simulink model "Semi_DP_1Hz"  (Simulink 8.7)
settings: Solver=ode4  StartTime=0.0  StopTime=12600  FixedStep=1  RelTol=1e-3
PreLoadFcn:
  | load('Initialization_data.mat');
undefined symbols (not defined in the file or in its folder): D, M, Ma, magnitude, P_mean, QTF_Dir, QTF_Freq, QTF_P, QTF_P1, QTF_Phase, QTF_T, RAO_Amp, RAO_Dir, RAO_Freq, RAO_Phase, RAO_Vel
libraries: simulink_extras x5, simulink x3
(part 1 of 2)
settings Model: Creator=Lither  LastModifiedBy=Administrator
settings OptimizationCC: ExpressionDepthLimit=2147483647
settings DebuggingCC: FcnCallInpInsideContextMsg=EnableAllAsWarning  StateNameClashWarn=warning
settings GRTTargetCC: CombineOutputUpdateFcns=off  GRTInterface=on
settings ConfigComp: CovSFcnEnable=off

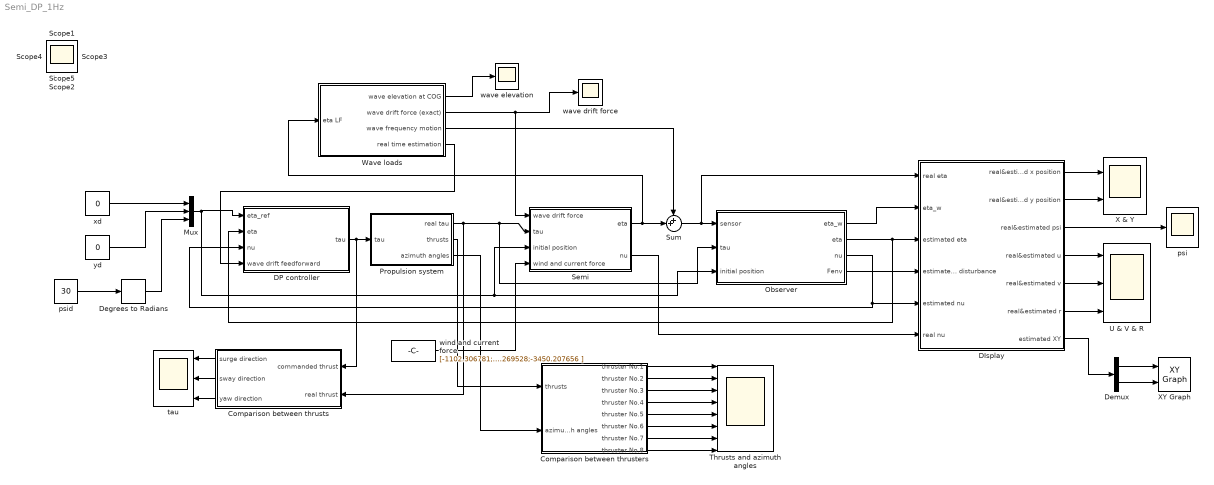
== system Semi_DP_1Hz ==
  Comparison between thrusters : Subsystem
  Comparison between thrusts : Subsystem
  DIsplay : Subsystem
  DP controller : Subsystem  mask(Nonlinear DP Controller){Kp=0.0015, Kd=0.06, Ki=1e-5, WFF_gain=0}
      mask prompts: Kp "Proportional Gain Matrix: Kp"; Kd "Derivative Gain Matrix: Kd"; Ki "Integral Gain Matrix: Ki"; WFF_gain "Wave feedforward Gain"
      mask help: PID controller for Set-Point Reulation in Surge, Sway and Yaw
      mask Help:
      | The nonlinear  PID controller uses the rotation matrix in yaw for proper scaling of the surge, sway and yaw gains as a function of the yaw angle.
      | INPUTS: (1) eta_ref, (2) eta, (3) nu. OUPUTS: (1) tau.
      mask Display: disp('PID controller')
  Degrees to Radians : simulink_extras/Transformations/Degrees to Radians
  Demux : Demux  Outputs=2
  Mux : Mux  Inputs=3
  Observer : Subsystem  mask(wave spectrum damping ratio){lambda=[0.0889 0.0839 0.1], w_o=[0.46 0.46 0.47], K3=5e5*diag([2 2 3500]), K4=6e5*diag([2 2 3500]), w_c=0.6, T=diag([10 10 10])}
      mask prompts: lambda "Relative damping ratio of wave spectrum: lambda"; w_o "Peak frequency of response spectrum: w_o (rad/s)"; K3 "Bias observer gain: K3"; K4 "Bias observer gain: K4"; w_c "Filter cut-off frequency: w_c (rad/s)"; T "Bias time constant: T (s)"
      mask init:
      | Zeta = 1;
      | Aw = blkdiag([0 1;-w_o(1)^2 -2*lambda(1)*w_o(1)],...
      |              [0 1;-w_o(2)^2 -2*lambda(2)*w_o(2)],...
      |              [0 1;-w_o(3)^2 -2*lambda(3)*w_o(3)]);
      | K1 = zeros(6,3);
      | for i =1:3
      |     K1(2*i-1,i) = -2*(Zeta - lambda(i))*w_c/w_o(i);
      |     K1(2*i,i) = 2*w_o(i)*(Zeta - lambda(i));
      | end
      | K2 = diag([w_c,w_c,w_c]);
      | Cw = zeros(3,6);
      | Cw(1,2) = 1;Cw(2,4) = 1;Cw(3,6) = 1;
      mask Display: disp('nonlinear passive observer')
  Propulsion system : Subsystem  mask{f0=[200;200;200;200;200;200;200;200], a0=[0;0;0;0;0;0;0;0], u0=[1; 1; 1; 1; 1; 1; 1; 1], wa=on}
      mask prompts: f0 "Initial values of thrusts"; a0 "Initial values of azimuth angles"; u0 "Thruster utilization"; wa "Show animation of thrust and azimuth angle"
  Semi : Subsystem  mask{wv=on}
      mask prompts: wv "Display animation of the vessel's motion"
  Sum : Sum  Inputs=++|
  Thrusts and azimuth angles : Scope  NumInputPorts=8
  U & V & R : Scope  NumInputPorts=3
  Wave loads : Subsystem
  X & Y : Scope  NumInputPorts=2
  XY Graph : simulink/Sinks/XY Graph  xmin=-20  xmax=20  ymin=-20  ymax=20  st=-1
  psi : Scope
  psid : Constant  Value=30
  tau : Scope  NumInputPorts=3
  wave drift force : Scope
  wave elevation : Scope
  wind and current force : Constant  Value=|
      | [-1102.306781;1391.269528;-3450.207656
      | ]
  xd : Constant  Value=0
  yd : Constant  Value=0
  Scope{,1..5} (6 alike) : Scope
  wires:
  xd/1 -> Mux/1
  yd/1 -> Mux/2
  Mux/1 -> Observer/3(initial position), Semi/3(initial position), DP controller/1(eta_ref)
  Semi/1(eta) -> Sum/2, Wave loads/1(eta LF)
  DP controller/1(tau) -> Propulsion system/1(tau), Comparison between thrusts/1(commanded thrust)
  Wave loads/2(wave drift force (exact)) -> Semi/1(wave drift force), wave drift force/1
  psid/1 -> Degrees to Radians/1
  Degrees to Radians/1 -> Mux/3
  Observer/3(nu) -> DP controller/3(nu), DIsplay/5(estimated nu)
  Observer/2(eta) -> DIsplay/3(estimated eta), DP controller/2(eta)
  Propulsion system/1(real tau) -> Comparison between thrusts/2(real thrust), Observer/2(tau), Semi/2(tau)
  Wave loads/1(wave elevation at COG) -> wave elevation/1
  Wave loads/3(wave frequency motion) -> Sum/1
  Sum/1 -> Observer/1(sensor), DIsplay/1(real eta)
  Comparison between thrusts/1(surge direction) -> tau/1
  Comparison between thrusts/2(sway direction) -> tau/2
  Comparison between thrusts/3(yaw direction) -> tau/3
  Propulsion system/2(thrusts) -> Comparison between thrusters/1(" thrusts")
  Propulsion system/3(azimuth angles) -> Comparison between thrusters/2(azimuth angles)
  Semi/2(nu) -> DIsplay/6(real nu)
  Observer/4(Fenv) -> DIsplay/4(estimated disturbance)
  DIsplay/1(real&estimated x position) -> X & Y/1
  DIsplay/2(real&estimated y position) -> X & Y/2
  DIsplay/3(real&estimated psi) -> psi/1
  DIsplay/4(real&estimated u) -> U & V & R/1
  DIsplay/5(real&estimated v) -> U & V & R/2
  Observer/1(eta_w) -> DIsplay/2(eta_w)
  DIsplay/6(real&estimated r) -> U & V & R/3
  wind and current force/1 -> Semi/4(wind and current force)
  Comparison between thrusters/1(thruster No.1) -> Thrusts and azimuth angles/1
  Comparison between thrusters/2(thruster No.2) -> Thrusts and azimuth angles/2
  Comparison between thrusters/8(thruster No.8) -> Thrusts and azimuth angles/8
  Comparison between thrusters/4(thruster No.4) -> Thrusts and azimuth angles/4
  Comparison between thrusters/6(thruster No.6) -> Thrusts and azimuth angles/6
  Comparison between thrusters/5(thruster No.5) -> Thrusts and azimuth angles/5
  Comparison between thrusters/3(thruster No.3) -> Thrusts and azimuth angles/3
  Comparison between thrusters/7(thruster No.7) -> Thrusts and azimuth angles/7
  Wave loads/4(real time estimation) -> DP controller/4(wave drift feedforward)
  Demux/1 -> XY Graph/1
  Demux/2 -> XY Graph/2
  DIsplay/7(estimated XY) -> Demux/1

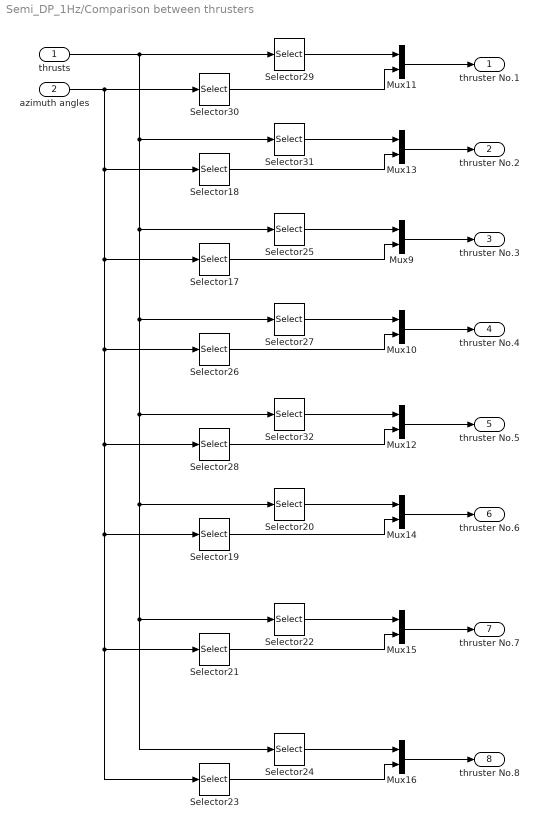
== system Semi_DP_1Hz/Comparison between thrusters ==
  " thrusts" : Inport
  azimuth angles : Inport  Port=2
  Mux{9..16} (8 alike) : Mux  Inputs=2
  Selector17 : Selector  InputPortWidth=8  IndexOptions=Index vector (dialog)  Indices=[3]  OutputSizes=1
  Selector18 : Selector  InputPortWidth=8  IndexOptions=Index vector (dialog)  Indices=[2]  OutputSizes=1
  Selector19 : Selector  InputPortWidth=8  IndexOptions=Index vector (dialog)  Indices=[6]  OutputSizes=1
  Selector20 : Selector  InputPortWidth=8  IndexOptions=Index vector (dialog)  Indices=[6]  OutputSizes=1
  Selector21 : Selector  InputPortWidth=8  IndexOptions=Index vector (dialog)  Indices=[7]  OutputSizes=1
  Selector22 : Selector  InputPortWidth=8  IndexOptions=Index vector (dialog)  Indices=[7]  OutputSizes=1
  Selector23 : Selector  InputPortWidth=8  IndexOptions=Index vector (dialog)  Indices=[8]  OutputSizes=1
  Selector24 : Selector  InputPortWidth=8  IndexOptions=Index vector (dialog)  Indices=[8]  OutputSizes=1
  Selector25 : Selector  InputPortWidth=8  IndexOptions=Index vector (dialog)  Indices=[3]  OutputSizes=1
  Selector26 : Selector  InputPortWidth=8  IndexOptions=Index vector (dialog)  Indices=[4]  OutputSizes=1
  Selector27 : Selector  InputPortWidth=8  IndexOptions=Index vector (dialog)  Indices=[4]  OutputSizes=1
  Selector28 : Selector  InputPortWidth=8  IndexOptions=Index vector (dialog)  Indices=[5]  OutputSizes=1
  Selector29 : Selector  InputPortWidth=8  IndexOptions=Index vector (dialog)  Indices=[1]  OutputSizes=1
  Selector30 : Selector  InputPortWidth=8  IndexOptions=Index vector (dialog)  Indices=[1]  OutputSizes=1
  Selector31 : Selector  InputPortWidth=8  IndexOptions=Index vector (dialog)  Indices=[2]  OutputSizes=1
  Selector32 : Selector  InputPortWidth=8  IndexOptions=Index vector (dialog)  Indices=[5]  OutputSizes=1
  thruster No.1 : Outport
  thruster No.2 : Outport  Port=2
  thruster No.3 : Outport  Port=3
  thruster No.4 : Outport  Port=4
  thruster No.5 : Outport  Port=5
  thruster No.6 : Outport  Port=6
  thruster No.7 : Outport  Port=7
  thruster No.8 : Outport  Port=8
  wires:
  Mux11/1 -> thruster No.1/1
  Selector29/1 -> Mux11/1
  Selector30/1 -> Mux11/2
  Selector31/1 -> Mux13/1
  Selector18/1 -> Mux13/2
  Mux13/1 -> thruster No.2/1
  " thrusts"/1 -> Selector29/1, Selector31/1, Selector25/1, Selector27/1, Selector32/1, Selector20/1, Selector22/1, Selector24/1
  Selector25/1 -> Mux9/1
  Selector17/1 -> Mux9/2
  Mux9/1 -> thruster No.3/1
  Selector27/1 -> Mux10/1
  Selector26/1 -> Mux10/2
  Selector32/1 -> Mux12/1
  Selector28/1 -> Mux12/2
  Selector20/1 -> Mux14/1
  Selector19/1 -> Mux14/2
  Mux10/1 -> thruster No.4/1
  Mux12/1 -> thruster No.5/1
  Mux14/1 -> thruster No.6/1
  azimuth angles/1 -> Selector30/1, Selector18/1, Selector17/1, Selector26/1, Selector28/1, Selector19/1, Selector23/1, Selector21/1
  Selector22/1 -> Mux15/1
  Selector21/1 -> Mux15/2
  Mux15/1 -> thruster No.7/1
  Selector24/1 -> Mux16/1
  Selector23/1 -> Mux16/2
  Mux16/1 -> thruster No.8/1

== system Semi_DP_1Hz/Comparison between thrusts ==
  commanded thrust : Inport
  real thrust : Inport  Port=2
  Mux3 : Mux  Inputs=2
  Mux5 : Mux  Inputs=2
  Mux6 : Mux  Inputs=2
  Selector10 : Selector  InputPortWidth=3  IndexOptions=Index vector (dialog)  Indices=[2]  OutputSizes=1
  Selector11 : Selector  InputPortWidth=3  IndexOptions=Index vector (dialog)  Indices=[3]  OutputSizes=1
  Selector6 : Selector  InputPortWidth=3  IndexOptions=Index vector (dialog)  Indices=[1]  OutputSizes=1
  Selector7 : Selector  InputPortWidth=3  IndexOptions=Index vector (dialog)  Indices=[1]  OutputSizes=1
  Selector8 : Selector  InputPortWidth=3  IndexOptions=Index vector (dialog)  Indices=[2]  OutputSizes=1
  Selector9 : Selector  InputPortWidth=3  IndexOptions=Index vector (dialog)  Indices=[3]  OutputSizes=1
  surge direction : Outport
  sway direction : Outport  Port=2
  yaw direction : Outport  Port=3
  wires:
  Selector9/1 -> Mux6/1
  Selector11/1 -> Mux6/2
  Selector10/1 -> Mux5/2
  Selector8/1 -> Mux5/1
  Selector7/1 -> Mux3/2
  Selector6/1 -> Mux3/1
  Mux3/1 -> surge direction/1
  Mux5/1 -> sway direction/1
  Mux6/1 -> yaw direction/1
  commanded thrust/1 -> Selector6/1, Selector8/1, Selector9/1
  real thrust/1 -> Selector7/1, Selector10/1, Selector11/1

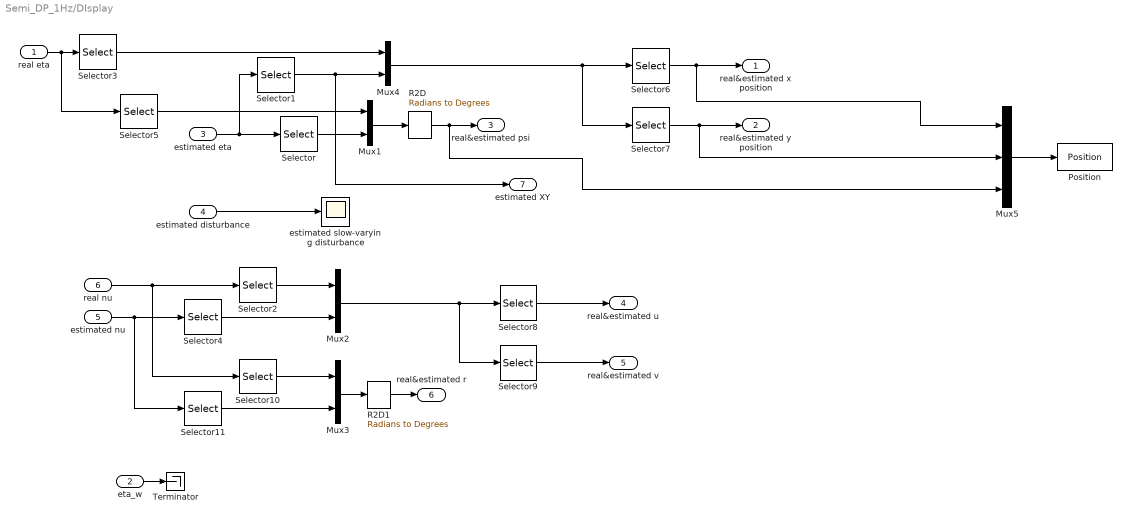
== system Semi_DP_1Hz/DIsplay ==
  real eta : Inport
  eta_w : Inport  Port=2
  estimated eta : Inport  Port=3
  estimated disturbance : Inport  Port=4
  estimated nu : Inport  Port=5
  real nu : Inport  Port=6
  Mux{1..4} (4 alike) : Mux  Inputs=2
  Mux5 : Mux  Inputs=3
  Position : ToWorkspace  VariableName=Position  SampleTime=-1
  R2D : simulink_extras/Transformations/Radians to Degrees
  R2D1 : simulink_extras/Transformations/Radians to Degrees
  Selector{,5,10..11} (4 alike) : Selector  InputPortWidth=3  IndexOptions=Index vector (dialog)  Indices=[3]  OutputSizes=1
  Selector{1..4} (4 alike) : Selector  InputPortWidth=3  IndexOptions=Index vector (dialog)  Indices=[1 2]  OutputSizes=1
  Selector6 : Selector  InputPortWidth=4  IndexOptions=Index vector (dialog)  Indices=[1 3]  OutputSizes=1
  Selector7 : Selector  InputPortWidth=4  IndexOptions=Index vector (dialog)  Indices=[2 4]  OutputSizes=1
  Selector8 : Selector  InputPortWidth=4  IndexOptions=Index vector (dialog)  Indices=[1 3]  OutputSizes=1
  Selector9 : Selector  InputPortWidth=4  IndexOptions=Index vector (dialog)  Indices=[2 4]  OutputSizes=1
  Terminator : Terminator
  estimated slow-varying disturbance : Scope
  real&estimated x position : Outport
  real&estimated y position : Outport  Port=2
  real&estimated psi : Outport  Port=3
  real&estimated u : Outport  Port=4
  real&estimated v : Outport  Port=5
  real&estimated r : Outport  Port=6
  estimated XY : Outport  Port=7
  wires:
  Selector/1 -> Mux1/2
  Mux1/1 -> R2D/1
  Selector1/1 -> estimated XY/1, Mux4/2
  Selector5/1 -> Mux1/1
  Selector2/1 -> Mux2/1
  Selector4/1 -> Mux2/2
  real eta/1 -> Selector3/1, Selector5/1
  estimated eta/1 -> Selector/1, Selector1/1
  real nu/1 -> Selector2/1, Selector10/1
  eta_w/1 -> Terminator/1
  estimated disturbance/1 -> estimated slow-varying disturbance/1
  Mux2/1 -> Selector8/1, Selector9/1
  estimated nu/1 -> Selector4/1, Selector11/1
  Mux4/1 -> Selector6/1, Selector7/1
  Selector8/1 -> real&estimated u/1
  Selector9/1 -> real&estimated v/1
  Mux3/1 -> R2D1/1
  R2D1/1 -> real&estimated r/1
  Selector10/1 -> Mux3/1
  Selector11/1 -> Mux3/2
  Selector3/1 -> Mux4/1
  R2D/1 -> Mux5/3, real&estimated psi/1
  Selector6/1 -> Mux5/1, real&estimated x position/1
  Selector7/1 -> Mux5/2, real&estimated y position/1
  Mux5/1 -> Position/1

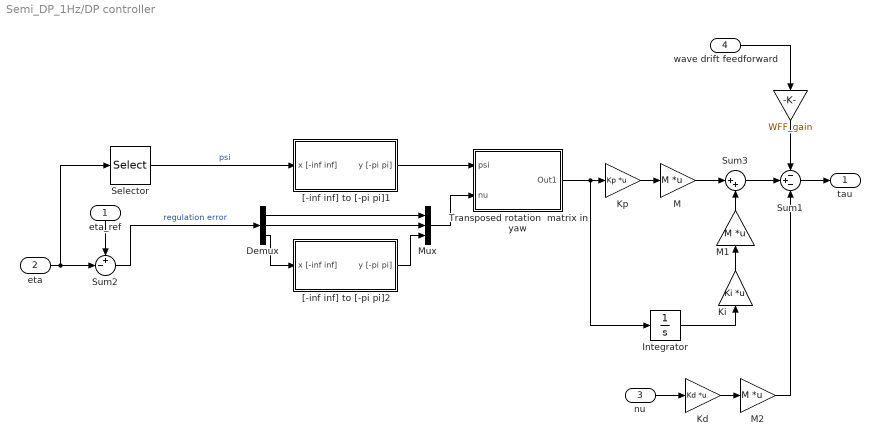
== system Semi_DP_1Hz/DP controller ==
  eta_ref : Inport
  eta : Inport  Port=2
  nu : Inport  Port=3
  wave drift feedforward : Inport  Port=4
  " " : Gain  Gain=WFF_gain  SaturateOnIntegerOverflow=on  OutDataTypeStr=Inherit: Same as input  ParamDataTypeStr=Inherit: Same as input
  Demux : Demux  Outputs=3
  Integrator : Integrator
  Kd : Gain  Gain=Kd  Multiplication=Matrix(K*u)  SaturateOnIntegerOverflow=on  OutDataTypeStr=Inherit: Same as input  ParamDataTypeStr=Inherit: Same as input
  Ki : Gain  Gain=Ki  Multiplication=Matrix(K*u)  SaturateOnIntegerOverflow=on  OutDataTypeStr=Inherit: Same as input  ParamDataTypeStr=Inherit: Same as input
  Kp : Gain  Gain=Kp  Multiplication=Matrix(K*u)  SaturateOnIntegerOverflow=on  OutDataTypeStr=Inherit: Same as input  ParamDataTypeStr=Inherit: Same as input
  M : Gain  Gain=M  Multiplication=Matrix(K*u)  SaturateOnIntegerOverflow=on  OutDataTypeStr=Inherit: Same as input  ParamDataTypeStr=Inherit: Same as input
  M1 : Gain  Gain=M  Multiplication=Matrix(K*u)  SaturateOnIntegerOverflow=on  OutDataTypeStr=Inherit: Same as input  ParamDataTypeStr=Inherit: Same as input
  M2 : Gain  Gain=M  Multiplication=Matrix(K*u)  SaturateOnIntegerOverflow=on  OutDataTypeStr=Inherit: Same as input  ParamDataTypeStr=Inherit: Same as input
  Mux : Mux  Inputs=3
  Selector : Selector  InputPortWidth=3  IndexOptions=Index vector (dialog)  Indices=[ 3]  OutputSizes=1
  Sum1 : Sum  Inputs=-+-  SaturateOnIntegerOverflow=on  InputSameDT=on  OutDataTypeStr=Inherit: Same as first input
  Sum2 : Sum  Inputs=+-|  SaturateOnIntegerOverflow=on  InputSameDT=on  OutDataTypeStr=Inherit: Same as first input
  Sum3 : Sum  Inputs=|++  SaturateOnIntegerOverflow=on  InputSameDT=on  OutDataTypeStr=Inherit: Same as first input
  Transposed rotation  matrix in yaw : Subsystem
  "[-inf inf] to [-pi pi]1" : Subsystem
  "[-inf inf] to [-pi pi]2" : Subsystem
  tau : Outport  InitialOutput=0
  wires:
  "[-inf inf] to [-pi pi]1"/1(y [-pi pi]) -> Transposed rotation  matrix in yaw/1(psi)
  Selector/1 -> "[-inf inf] to [-pi pi]1"/1(x [-inf inf])  "psi"
  Mux/1 -> Transposed rotation  matrix in yaw/2(nu)
  Demux/1 -> Mux/1
  Demux/2 -> Mux/2
  "[-inf inf] to [-pi pi]2"/1(y [-pi pi]) -> Mux/3
  Sum2/1 -> Demux/1  "regulation error"
  Demux/3 -> "[-inf inf] to [-pi pi]2"/1(x [-inf inf])
  eta_ref/1 -> Sum2/1
  Sum1/1 -> tau/1
  eta/1 -> Sum2/2, Selector/1
  nu/1 -> Kd/1
  Integrator/1 -> Ki/1
  Kp/1 -> M/1
  Ki/1 -> M1/1
  Transposed rotation  matrix in yaw/1(Out1) -> Kp/1, Integrator/1
  Kd/1 -> M2/1
  M/1 -> Sum3/1
  M1/1 -> Sum3/2
  wave drift feedforward/1 -> " "/1
  " "/1 -> Sum1/1
  M2/1 -> Sum1/3
  Sum3/1 -> Sum1/2

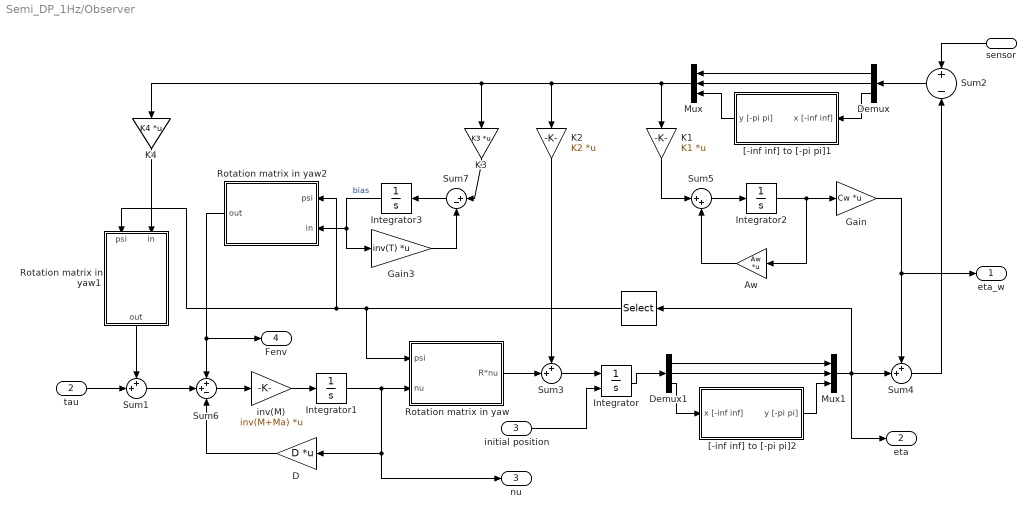
== system Semi_DP_1Hz/Observer ==
  sensor : Inport
  tau : Inport  Port=2
  initial position : Inport  Port=3
  " " : Selector  InputPortWidth=3  IndexOptions=Index vector (dialog)  Indices=[3]  OutputSizes=1
  Aw : Gain  Gain=Aw  Multiplication=Matrix(K*u)  SaturateOnIntegerOverflow=on  OutDataTypeStr=Inherit: Same as input  ParamDataTypeStr=Inherit: Same as input
  D : Gain  Gain=D  Multiplication=Matrix(K*u)  SaturateOnIntegerOverflow=on  OutDataTypeStr=Inherit: Same as input  ParamDataTypeStr=Inherit: Same as input
  Demux : Demux  Outputs=3
  Demux1 : Demux  Outputs=3
  Gain : Gain  Gain=Cw  Multiplication=Matrix(K*u)
  Gain3 : Gain  Gain=inv(T)  Multiplication=Matrix(K*u)  SaturateOnIntegerOverflow=on  OutDataTypeStr=Inherit: Same as input  ParamDataTypeStr=Inherit: Same as input
  Integrator : Integrator  InitialConditionSource=external
  Integrator1 : Integrator
  Integrator2 : Integrator
  Integrator3 : Integrator
  K1 : Gain  Gain=K1  Multiplication=Matrix(K*u)  SaturateOnIntegerOverflow=on  OutDataTypeStr=Inherit: Same as input  ParamDataTypeStr=Inherit: Same as input
  K2 : Gain  Gain=K2  Multiplication=Matrix(K*u)  SaturateOnIntegerOverflow=on  OutDataTypeStr=Inherit: Same as input  ParamDataTypeStr=Inherit: Same as input
  K3 : Gain  Gain=K3  Multiplication=Matrix(K*u)  SaturateOnIntegerOverflow=on  OutDataTypeStr=Inherit: Same as input  ParamDataTypeStr=Inherit: Same as input
  K4 : Gain  Gain=K4  Multiplication=Matrix(K*u)  SaturateOnIntegerOverflow=on  OutDataTypeStr=Inherit: Same as input  ParamDataTypeStr=Inherit: Same as input
  Mux : Mux  Inputs=3
  Mux1 : Mux  Inputs=3
  Rotation matrix in yaw : Subsystem
  Rotation matrix in yaw1 : Subsystem
  Rotation matrix in yaw2 : Subsystem
  Sum1 : Sum  Inputs=++|  SaturateOnIntegerOverflow=on  InputSameDT=on  OutDataTypeStr=Inherit: Same as first input
  Sum2 : Sum  Inputs=+|-  SaturateOnIntegerOverflow=on  InputSameDT=on  OutDataTypeStr=Inherit: Same as first input
  Sum3 : Sum  Inputs=++|  SaturateOnIntegerOverflow=on  InputSameDT=on  OutDataTypeStr=Inherit: Same as first input
  Sum4 : Sum  Inputs=++|  SaturateOnIntegerOverflow=on  InputSameDT=on  OutDataTypeStr=Inherit: Same as first input
  Sum5 : Sum  Inputs=|++  SaturateOnIntegerOverflow=on  InputSameDT=on  OutDataTypeStr=Inherit: Same as first input
  Sum6 : Sum  Inputs=++-  SaturateOnIntegerOverflow=on  InputSameDT=on  OutDataTypeStr=Inherit: Same as first input
  Sum7 : Sum  Inputs=|+-  SaturateOnIntegerOverflow=on  InputSameDT=on  OutDataTypeStr=Inherit: Same as first input
  "[-inf inf] to [-pi pi]1" : Subsystem  mask([-inf inf] to [-pi pi]){}
      mask help: Converts an angle in rad to (-pi pi)
  "[-inf inf] to [-pi pi]2" : Subsystem
  inv(M) : Gain  Gain=inv(M+Ma)  Multiplication=Matrix(K*u)  SaturateOnIntegerOverflow=on  OutDataTypeStr=Inherit: Same as input  ParamDataTypeStr=Inherit: Same as input
  eta_w : Outport
  eta : Outport  Port=2
  nu : Outport  Port=3
  Fenv : Outport  Port=4
  wires:
  tau/1 -> Sum1/2
  sensor/1 -> Sum2/1
  Gain3/1 -> Sum7/2
  Sum7/1 -> Integrator3/1
  Integrator3/1 -> Gain3/1, Rotation matrix in yaw2/2(in)  "bias"
  Sum4/1 -> Sum2/2
  Integrator/1 -> Demux1/1
  Sum3/1 -> Integrator/1
  Sum2/1 -> Demux/1
  Demux/3 -> "[-inf inf] to [-pi pi]1"/1(x [-inf inf])
  "[-inf inf] to [-pi pi]1"/1(y [-pi pi]) -> Mux/3
  Demux/1 -> Mux/1
  Demux/2 -> Mux/2
  Mux/1 -> K1/1, K2/1, K4/1, K3/1
  Demux1/1 -> Mux1/1
  Demux1/2 -> Mux1/2
  "[-inf inf] to [-pi pi]2"/1(y [-pi pi]) -> Mux1/3
  Demux1/3 -> "[-inf inf] to [-pi pi]2"/1(x [-inf inf])
  Mux1/1 -> eta/1, Sum4/2, " "/1
  Sum5/1 -> Integrator2/1
  K1/1 -> Sum5/1
  Integrator2/1 -> Gain/1, Aw/1
  Aw/1 -> Sum5/2
  K2/1 -> Sum3/1
  Rotation matrix in yaw/1(R*nu) -> Sum3/2
  K3/1 -> Sum7/1
  inv(M)/1 -> Integrator1/1
  Sum6/1 -> inv(M)/1
  Integrator1/1 -> Rotation matrix in yaw/2(nu), D/1, nu/1
  " "/1 -> Rotation matrix in yaw/1(psi), Rotation matrix in yaw1/1(psi), Rotation matrix in yaw2/1(psi)
  Sum1/1 -> Sum6/2
  D/1 -> Sum6/3
  K4/1 -> Rotation matrix in yaw1/2(in)
  Rotation matrix in yaw1/1(out) -> Sum1/1
  Rotation matrix in yaw2/1(out) -> Sum6/1, Fenv/1
  initial position/1 -> Integrator/2
  Gain/1 -> Sum4/1, eta_w/1

== system Semi_DP_1Hz/Propulsion system ==
  tau : Inport
  AzimuthAngle : ToWorkspace  VariableName=AziAng  SampleTime=-1
  Gain : Gain  Gain=1/1000
  Gain1 : Gain  Gain=1000
  Level-2 MATLAB S-Function : M-S-Function  FunctionName=msfunTA_PA  Parameters=f0,a0,wa,u0
  RealTau : ToWorkspace  VariableName=RealTau  SampleTime=-1
  Terminator : Terminator
  Terminator1 : Terminator
  Terminator2 : Terminator
  ThrusterForce : ToWorkspace  VariableName=Thrust  SampleTime=-1
  real tau : Outport
  thrusts : Outport  Port=2
  azimuth angles : Outport  Port=3
  wires:
  tau/1 -> Gain/1
  Level-2 MATLAB S-Function/2 -> Terminator/1
  Level-2 MATLAB S-Function/3 -> AzimuthAngle/1, azimuth angles/1
  Level-2 MATLAB S-Function/4 -> Terminator1/1
  Level-2 MATLAB S-Function/5 -> Gain1/1
  Level-2 MATLAB S-Function/6 -> Terminator2/1
  Level-2 MATLAB S-Function/1 -> ThrusterForce/1, thrusts/1
  Gain/1 -> Level-2 MATLAB S-Function/1
  Gain1/1 -> RealTau/1, real tau/1

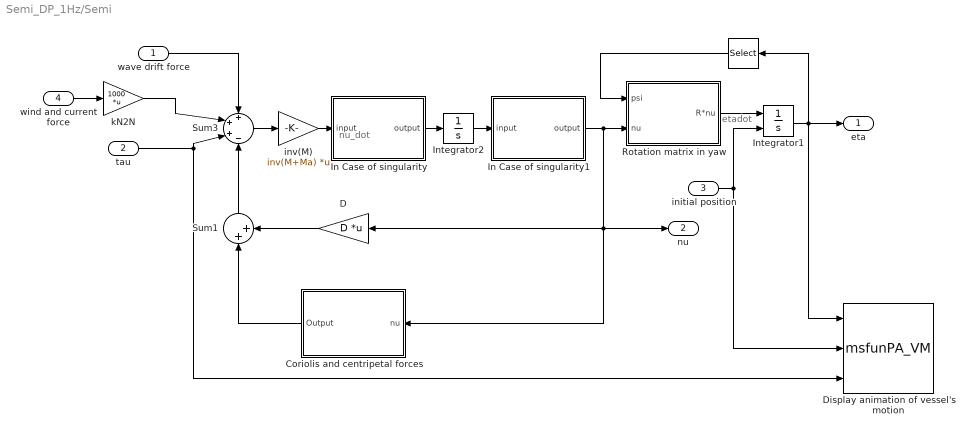
== system Semi_DP_1Hz/Semi ==
  note: nu_dot
  note: etadot
  wave drift force : Inport
  tau : Inport  Port=2
  initial position : Inport  Port=3
  wind and current force : Inport  Port=4
  " " : Selector  InputPortWidth=3  IndexOptions=Index vector (dialog)  Indices=[3]  OutputSizes=1
  Coriolis and centripetal forces : Subsystem
  D : Gain  Gain=D  Multiplication=Matrix(K*u)  SaturateOnIntegerOverflow=on  OutDataTypeStr=Inherit: Same as input  ParamDataTypeStr=Inherit: Same as input
  Display animation of vessel's motion : M-S-Function  FunctionName=msfunPA_VM  Parameters=wv
  In Case of singularity : Subsystem
  In Case of singularity1 : Subsystem
  Integrator1 : Integrator  InitialConditionSource=external  InitialCondition=1.05
  Integrator2 : Integrator
  Rotation matrix in yaw : Subsystem
  Sum1 : Sum  Inputs=|++  SaturateOnIntegerOverflow=on  InputSameDT=on  OutDataTypeStr=Inherit: Same as first input
  Sum3 : Sum  Inputs=+++-  SaturateOnIntegerOverflow=on  InputSameDT=on  OutDataTypeStr=Inherit: Same as first input
  inv(M) : Gain  Gain=inv(M+Ma)  Multiplication=Matrix(K*u)  SaturateOnIntegerOverflow=on  OutDataTypeStr=Inherit: Same as input  ParamDataTypeStr=Inherit: Same as input
  kN2N : Gain  Gain=1000  Multiplication=Matrix(K*u)  SaturateOnIntegerOverflow=on  OutDataTypeStr=Inherit: Same as input  ParamDataTypeStr=Inherit: Same as input
  eta : Outport
  nu : Outport  Port=2
  wires:
  Sum3/1 -> inv(M)/1
  inv(M)/1 -> In Case of singularity/1(input)
  Rotation matrix in yaw/1(R*nu) -> Integrator1/1
  Integrator1/1 -> eta/1, " "/1, Display animation of vessel's motion/1
  " "/1 -> Rotation matrix in yaw/1(psi)
  tau/1 -> Display animation of vessel's motion/3, Sum3/3
  initial position/1 -> Integrator1/2, Display animation of vessel's motion/2
  Sum1/1 -> Sum3/4
  wind and current force/1 -> kN2N/1
  Integrator2/1 -> In Case of singularity1/1(input)
  In Case of singularity/1(output) -> Integrator2/1
  In Case of singularity1/1(output) -> Rotation matrix in yaw/2(nu), D/1, Coriolis and centripetal forces/1(nu), nu/1
  wave drift force/1 -> Sum3/1
  D/1 -> Sum1/2
  Coriolis and centripetal forces/1(Output) -> Sum1/1
  kN2N/1 -> Sum3/2

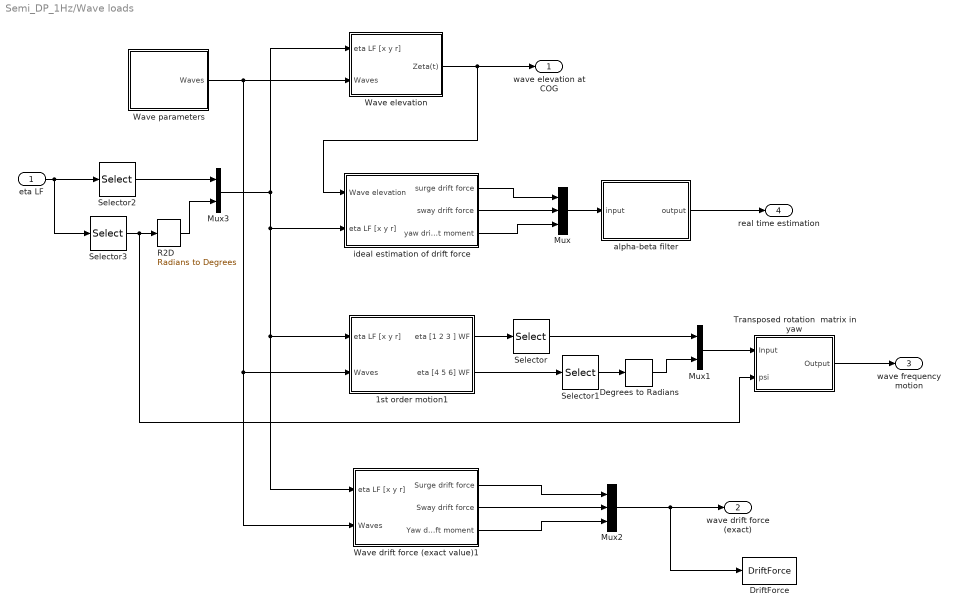
== system Semi_DP_1Hz/Wave loads ==
  eta LF : Inport
  1st order motion1 : Subsystem  mask(Motion RAO){}
      mask help: Calculate the wave-frequency motion of a vessel in 6 DOF from its RAOs and a sea state defined by a set of harmonic waves.
  Degrees to Radians : simulink_extras/Transformations/Degrees to Radians
  DriftForce : ToWorkspace  VariableName=DriftForce  SampleTime=-1
  Mux : Mux  Inputs=3
  Mux1 : Mux  Inputs=2
  Mux2 : Mux  Inputs=3
  Mux3 : Mux  Inputs=2
  R2D : simulink_extras/Transformations/Radians to Degrees
  Selector : Selector  InputPortWidth=3  IndexOptions=Index vector (dialog)  Indices=[1 2]  OutputSizes=1
  Selector1 : Selector  InputPortWidth=3  IndexOptions=Index vector (dialog)  Indices=[3]  OutputSizes=1
  Selector2 : Selector  InputPortWidth=3  IndexOptions=Index vector (dialog)  Indices=[1 2]  OutputSizes=1
  Selector3 : Selector  InputPortWidth=3  IndexOptions=Index vector (dialog)  Indices=[3]  OutputSizes=1
  Transposed rotation  matrix in yaw : Subsystem
  Wave drift force (exact value)1 : Subsystem  mask(Wave drift force (exact value based on full QTF matrix)){}
      mask help: Calculate the mean and slow varying wave drift forces based on full QTF matrix.
  Wave elevation : Subsystem  mask(Wave elevation){}
      mask help: Caclulates wave surface elevation Zeta at the point [x y].
  Wave parameters : Subsystem  mask(JONSWAP Spectrum Generator){Hs=5.27, Tp=13.4, gamma=3.3, nfr=200, displayplots=off, Zeta_a=0, Omega=0, Phase=0, Wavenum=0}
      mask prompts: Hs "Significant wave height Hs (m)"; Tp "Peak period (s)"; gamma "Spectrum peakedness factor"; nfr "Number of frequencies"; displayplots "Display plot"; Zeta_a "Amplitude vector 'Zeta_a' (m)"; Omega "Frequency vector 'Omega' (rad/s)"; Phase "Phase vector 'Phase' (rad)"; Wavenum "Wave number vector 'Wavenum' (1/m)"
      mask help: Generate long-crested irregular waves based on JONSWAP spectrum
      mask init:
      | [Omega,Zeta_a,Wavenum,Phase]=jonspec_fixed(Hs,Tp,gamma,nfr,displayplots);
  alpha-beta filter : Subsystem  mask(alpha-beta filter){a=8e-2, b=1e-12}
      mask prompts: a "alpha"; b "beta"
  "ideal estimation of drift force " : Subsystem  mask(Estimate the second order wave force in real time){}
      mask help: The real-time estimation of wave drift force is based on the mean value of QTF_P on the diagonal and wave elevation.
  wave elevation at COG : Outport
  wave drift force (exact) : Outport  Port=2
  wave frequency motion : Outport  Port=3
  real time estimation : Outport  Port=4
  wires:
  Wave elevation/1(Zeta(t)) -> "ideal estimation of drift force "/1(Wave elevation), wave elevation at COG/1
  Wave parameters/1(Waves) -> Wave elevation/2(Waves), Wave drift force (exact value)1/2(Waves), 1st order motion1/2(Waves)
  eta LF/1 -> Selector2/1, Selector3/1
  1st order motion1/1(eta [1 2 3 ] WF) -> Selector/1
  Selector/1 -> Mux1/1
  1st order motion1/2(eta [4 5 6] WF) -> Selector1/1
  Selector1/1 -> Degrees to Radians/1
  Mux1/1 -> Transposed rotation  matrix in yaw/1(Input)
  Wave drift force (exact value)1/2(Sway drift force) -> Mux2/2
  Wave drift force (exact value)1/3(Yaw drift moment) -> Mux2/3
  Wave drift force (exact value)1/1(Surge drift force) -> Mux2/1
  Selector3/1 -> R2D/1, Transposed rotation  matrix in yaw/2(psi)
  Selector2/1 -> Mux3/1
  R2D/1 -> Mux3/2
  Mux3/1 -> "ideal estimation of drift force "/2(eta LF [x y r]), Wave drift force (exact value)1/1(eta LF [x y r]), 1st order motion1/1(eta LF [x y r]), Wave elevation/1(eta LF [x y r])
  Degrees to Radians/1 -> Mux1/2
  Transposed rotation  matrix in yaw/1(Output) -> wave frequency motion/1
  "ideal estimation of drift force "/1(surge drift force) -> Mux/1
  "ideal estimation of drift force "/2(sway drift force) -> Mux/2
  Mux/1 -> alpha-beta filter/1(input)
  "ideal estimation of drift force "/3(yaw drift moment) -> Mux/3
  Mux2/1 -> DriftForce/1, wave drift force (exact)/1
  alpha-beta filter/1(output) -> real time estimation/1

== system Semi_DP_1Hz/DP controller/Transposed rotation  matrix in yaw ==
  psi : Inport
  nu : Inport  Port=2
  Mux : Mux  Inputs=2
  Mux1 : Mux  Inputs=3
  Row1 : Fcn  Expr=cos(u(1))*u(2)+sin(u(1))*u(3)
  Row2 : Fcn  Expr=-sin(u(1))*u(2)+cos(u(1))*u(3)
  Row3 : Fcn  Expr=u(4)
  Out1 : Outport
  wires:
  Mux/1 -> Row3/1, Row2/1, Row1/1
  Row1/1 -> Mux1/1
  Row2/1 -> Mux1/2
  Row3/1 -> Mux1/3
  Mux1/1 -> Out1/1
  psi/1 -> Mux/1
  nu/1 -> Mux/2

== system Semi_DP_1Hz/DP controller/[-inf inf] to [-pi pi]1 ==
  note: x
  note: r
  x [-inf inf] : Inport
  Constant : Constant  Value=2*pi
  Gain : Gain  Gain=pi  SaturateOnIntegerOverflow=on  OutDataTypeStr=Inherit: Same as input  ParamDataTypeStr=Inherit: Same as input
  Math Function : Math  Operator=rem  SaturateOnIntegerOverflow=on
  Saturation : Saturate  UpperLimit=1e10  LowerLimit=-1e10
  Sign : Signum
  Sum : Sum  Inputs=|+-  SaturateOnIntegerOverflow=on
  Sum1 : Sum  Inputs=|++  SaturateOnIntegerOverflow=on
  y [-pi pi] : Outport
  wires:
  x [-inf inf]/1 -> Saturation/1
  Sign/1 -> Gain/1
  Gain/1 -> Sum/2, Sum1/2
  Sum1/1 -> Math Function/1
  Constant/1 -> Math Function/2
  Math Function/1 -> Sum/1
  Sum/1 -> y [-pi pi]/1
  Saturation/1 -> Sum1/1, Sign/1

== system Semi_DP_1Hz/DP controller/[-inf inf] to [-pi pi]2 ==
  note: r
  note: x
  x [-inf inf] : Inport
  Constant : Constant  Value=2*pi
  Gain : Gain  Gain=pi  SaturateOnIntegerOverflow=on  OutDataTypeStr=Inherit: Same as input  ParamDataTypeStr=Inherit: Same as input
  Math Function : Math  Operator=rem  SaturateOnIntegerOverflow=on
  Saturation : Saturate  UpperLimit=1e10  LowerLimit=-1e10
  Sign : Signum
  Sum : Sum  Inputs=|+-  SaturateOnIntegerOverflow=on
  Sum1 : Sum  Inputs=|++  SaturateOnIntegerOverflow=on
  y [-pi pi] : Outport
  wires:
  Saturation/1 -> Sign/1, Sum1/1
  Sum/1 -> y [-pi pi]/1
  Math Function/1 -> Sum/1
  Constant/1 -> Math Function/2
  Sum1/1 -> Math Function/1
  Gain/1 -> Sum1/2, Sum/2
  Sign/1 -> Gain/1
  x [-inf inf]/1 -> Saturation/1

== system Semi_DP_1Hz/Observer/Rotation matrix in yaw ==
  psi : Inport
  nu : Inport  Port=2
  Fcn : Fcn  Expr=cos(u(1))*u(2)-sin(u(1))*u(3)
  Fcn1 : Fcn  Expr=sin(u(1))*u(2)+cos(u(1))*u(3)
  Fcn2 : Fcn  Expr=u(4)
  Mux : Mux  Inputs=2
  Mux1 : Mux  Inputs=3
  R*nu : Outport
  wires:
  Mux1/1 -> R*nu/1  "eta_dot"
  Mux/1 -> Fcn/1, Fcn1/1, Fcn2/1
  psi/1 -> Mux/1
  nu/1 -> Mux/2
  Fcn1/1 -> Mux1/2  "y_dot"
  Fcn/1 -> Mux1/1  "x_dot"
  Fcn2/1 -> Mux1/3  "psi_dot"

== system Semi_DP_1Hz/Observer/Rotation matrix in yaw1 ==
  psi : Inport
  in : Inport  Port=2
  Fcn : Fcn  Expr=cos(u(1))*u(2)+sin(u(1))*u(3)
  Fcn1 : Fcn  Expr=-sin(u(1))*u(2)+cos(u(1))*u(3)
  Fcn2 : Fcn  Expr=u(4)
  Mux : Mux  Inputs=2
  Mux1 : Mux  Inputs=3
  out : Outport
  wires:
  Fcn2/1 -> Mux1/3
  Fcn/1 -> Mux1/1
  Fcn1/1 -> Mux1/2
  in/1 -> Mux/2
  psi/1 -> Mux/1
  Mux/1 -> Fcn2/1, Fcn1/1, Fcn/1
  Mux1/1 -> out/1

== system Semi_DP_1Hz/Observer/Rotation matrix in yaw2 ==
  psi : Inport
  in : Inport  Port=2
  Fcn : Fcn  Expr=cos(u(1))*u(2)+sin(u(1))*u(3)
  Fcn1 : Fcn  Expr=-sin(u(1))*u(2)+cos(u(1))*u(3)
  Fcn2 : Fcn  Expr=u(4)
  Mux : Mux  Inputs=2
  Mux1 : Mux  Inputs=3
  out : Outport
  wires:
  Mux1/1 -> out/1
  Mux/1 -> Fcn/1, Fcn1/1, Fcn2/1
  psi/1 -> Mux/1
  in/1 -> Mux/2
  Fcn1/1 -> Mux1/2
  Fcn/1 -> Mux1/1
  Fcn2/1 -> Mux1/3

== system Semi_DP_1Hz/Observer/[-inf inf] to [-pi pi]1 ==
  note: x
  note: r
  x [-inf inf] : Inport
  Constant : Constant  Value=2*pi
  Gain : Gain  Gain=pi  SaturateOnIntegerOverflow=on  OutDataTypeStr=Inherit: Same as input  ParamDataTypeStr=Inherit: Same as input
  Math Function : Math  Operator=rem  SaturateOnIntegerOverflow=on
  Saturation : Saturate  UpperLimit=1e10  LowerLimit=-1e10
  Sign : Signum
  Sum : Sum  Inputs=|+-  SaturateOnIntegerOverflow=on
  Sum1 : Sum  Inputs=|++  SaturateOnIntegerOverflow=on
  y [-pi pi] : Outport
  wires:
  x [-inf inf]/1 -> Saturation/1
  Sign/1 -> Gain/1
  Gain/1 -> Sum/2, Sum1/2
  Sum1/1 -> Math Function/1
  Constant/1 -> Math Function/2
  Math Function/1 -> Sum/1
  Sum/1 -> y [-pi pi]/1
  Saturation/1 -> Sum1/1, Sign/1

== system Semi_DP_1Hz/Observer/[-inf inf] to [-pi pi]2 ==
  note: r
  note: x
  x [-inf inf] : Inport
  Constant : Constant  Value=2*pi
  Gain : Gain  Gain=pi  SaturateOnIntegerOverflow=on  OutDataTypeStr=Inherit: Same as input  ParamDataTypeStr=Inherit: Same as input
  Math Function : Math  Operator=rem  SaturateOnIntegerOverflow=on
  Saturation : Saturate  UpperLimit=1e10  LowerLimit=-1e10
  Sign : Signum
  Sum : Sum  Inputs=|+-  SaturateOnIntegerOverflow=on
  Sum1 : Sum  Inputs=|++  SaturateOnIntegerOverflow=on
  y [-pi pi] : Outport
  wires:
  Saturation/1 -> Sign/1, Sum1/1
  Sum/1 -> y [-pi pi]/1
  Math Function/1 -> Sum/1
  Constant/1 -> Math Function/2
  Sum1/1 -> Math Function/1
  Gain/1 -> Sum1/2, Sum/2
  Sign/1 -> Gain/1
  x [-inf inf]/1 -> Saturation/1

== system Semi_DP_1Hz/Semi/Coriolis and centripetal forces ==
  nu : Inport
  Mux : Mux  Inputs=3
  Selector1 : Selector  InputPortWidth=3  IndexOptions=Index vector (dialog)  Indices=[1 ]  OutputSizes=1
  Selector2 : Selector  InputPortWidth=3  IndexOptions=Index vector (dialog)  Indices=[2]  OutputSizes=1
  Selector3 : Selector  InputPortWidth=3  IndexOptions=Index vector (dialog)  Indices=[3]  OutputSizes=1
  Subsystem : Subsystem
  Subsystem1 : Subsystem
  Subsystem2 : Subsystem
  Output : Outport
  wires:
  nu/1 -> Selector1/1, Selector2/1, Selector3/1
  Selector2/1 -> Subsystem/1(v), Subsystem2/2(v)  "v"
  Selector3/1 -> Subsystem/2(r), Subsystem1/2(r), Subsystem2/3(r)  "r"
  Selector1/1 -> Subsystem1/1(u), Subsystem2/1(u)  "u"
  Subsystem/1(x direction) -> Mux/1
  Subsystem1/1(y direction) -> Mux/2
  Subsystem2/1(yaw direction) -> Mux/3
  Mux/1 -> Output/1

== system Semi_DP_1Hz/Semi/In Case of singularity ==
  input : Inport
  Compare To Constant : simulink/Logic and Bit Operations/Compare To Constant  relop=>=  const=1e8  OutDataTypeStr=boolean
  Stop Simulation : Stop
  output : Outport
  wires:
  input/1 -> output/1, Compare To Constant/1
  Compare To Constant/1 -> Stop Simulation/1

== system Semi_DP_1Hz/Semi/In Case of singularity1 ==
  input : Inport
  Compare To Constant : simulink/Logic and Bit Operations/Compare To Constant  relop=>=  const=1e10  OutDataTypeStr=boolean
  Stop Simulation : Stop
  output : Outport
  wires:
  input/1 -> output/1, Compare To Constant/1
  Compare To Constant/1 -> Stop Simulation/1

== system Semi_DP_1Hz/Semi/Rotation matrix in yaw ==
  psi : Inport
  nu : Inport  Port=2
  Fcn : Fcn  Expr=cos(u(1))*u(2)-sin(u(1))*u(3)
  Fcn1 : Fcn  Expr=sin(u(1))*u(2)+cos(u(1))*u(3)
  Fcn2 : Fcn  Expr=u(4)
  Mux : Mux  Inputs=2
  Mux1 : Mux  Inputs=3
  R*nu : Outport
  wires:
  Mux1/1 -> R*nu/1  "eta_dot"
  Mux/1 -> Fcn/1, Fcn1/1, Fcn2/1
  psi/1 -> Mux/1
  nu/1 -> Mux/2
  Fcn1/1 -> Mux1/2  "y_dot"
  Fcn/1 -> Mux1/1  "x_dot"
  Fcn2/1 -> Mux1/3  "psi_dot"

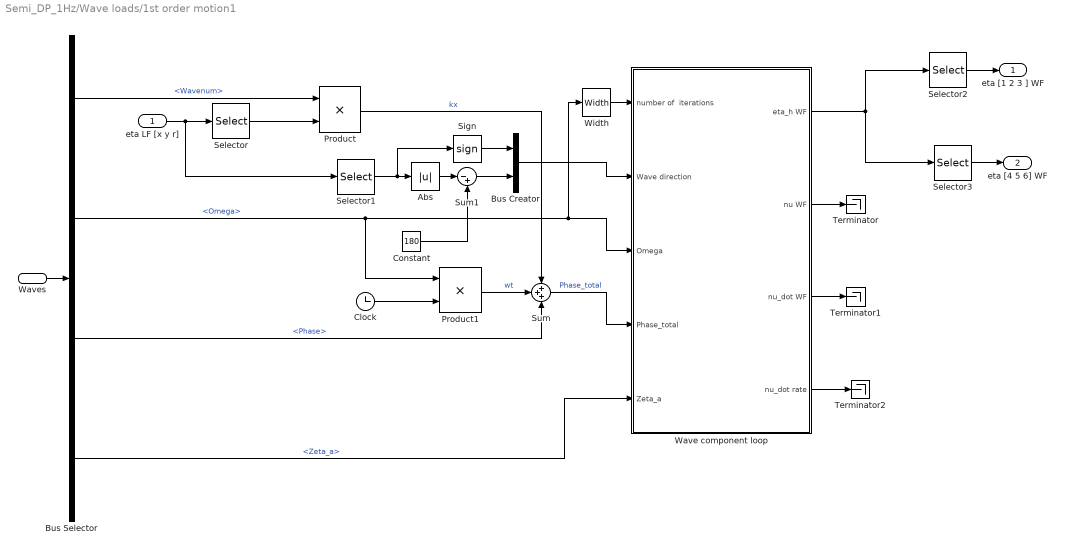
== system Semi_DP_1Hz/Wave loads/1st order motion1 ==
  eta LF [x y r] : Inport
  Waves : Inport  Port=2
  Abs : Abs
  Bus Creator : BusCreator  Inputs=2
  Bus Selector : BusSelector  OutputSignals=Wavenum,Omega,Phase,Zeta_a
  Clock : Clock
  Constant : Constant  Value=180
  Product : Product  Inputs=**  SaturateOnIntegerOverflow=on  OutDataTypeStr=Inherit: Same as first input
  Product1 : Product  Inputs=**  SaturateOnIntegerOverflow=on  OutDataTypeStr=Inherit: Same as first input
  Selector : Selector  InputPortWidth=3  IndexOptions=Index vector (dialog)  Indices=1  OutputSizes=1
  Selector1 : Selector  InputPortWidth=3  IndexOptions=Index vector (dialog)  Indices=3  OutputSizes=1
  Selector2 : Selector  InputPortWidth=6  IndexOptions=Index vector (dialog)  Indices=[1 2 3]  OutputSizes=1
  Selector3 : Selector  InputPortWidth=6  IndexOptions=Index vector (dialog)  Indices=[4 5 6]  OutputSizes=1
  Sign : Signum
  Sum : Sum  Inputs=+++  SaturateOnIntegerOverflow=on
  Sum1 : Sum  Inputs=|-+
  Terminator : Terminator
  Terminator1 : Terminator
  Terminator2 : Terminator
  Wave component loop : Subsystem  TreatAsAtomicUnit=on
  Width : Width  DataType=int32
  eta [1 2 3 ] WF : Outport
  eta [4 5 6] WF : Outport  Port=2
  wires:
  Wave component loop/1(eta_h WF) -> Selector2/1, Selector3/1
  Selector3/1 -> eta [4 5 6] WF/1
  Bus Creator/1 -> Wave component loop/2(Wave direction)
  Sum1/1 -> Bus Creator/2
  Sign/1 -> Bus Creator/1
  Abs/1 -> Sum1/1
  Selector1/1 -> Sign/1, Abs/1
  Constant/1 -> Sum1/2
  eta LF [x y r]/1 -> Selector1/1, Selector/1
  Bus Selector/1 -> Product/1  "<Wavenum>"
  Selector/1 -> Product/2
  Selector2/1 -> eta [1 2 3 ] WF/1
  Wave component loop/4(nu_dot rate) -> Terminator2/1
  Bus Selector/3 -> Sum/3  "<Phase>"
  Waves/1 -> Bus Selector/1
  Product1/1 -> Sum/2  "wt"
  Clock/1 -> Product1/2
  Bus Selector/2 -> Width/1, Wave component loop/3(Omega), Product1/1  "<Omega>"
  Sum/1 -> Wave component loop/4(Phase_total)  "Phase_total"
  Bus Selector/4 -> Wave component loop/5(Zeta_a)  "<Zeta_a>"
  Width/1 -> Wave component loop/1(number of  iterations)
  Wave component loop/2(nu WF) -> Terminator/1
  Wave component loop/3(nu_dot WF) -> Terminator1/1
  Product/1 -> Sum/1  "kx"

== system Semi_DP_1Hz/Wave loads/Transposed rotation  matrix in yaw ==
  Input : Inport
  psi : Inport  Port=2
  Mux : Mux  Inputs=2
  Mux1 : Mux  Inputs=3
  Row1 : Fcn  Expr=cos(u(1))*u(2)-sin(u(1))*u(3)
  Row2 : Fcn  Expr=sin(u(1))*u(2)+cos(u(1))*u(3)
  Row3 : Fcn  Expr=u(4)
  Output : Outport
  wires:
  Mux/1 -> Row3/1, Row2/1, Row1/1
  Row1/1 -> Mux1/1
  Row2/1 -> Mux1/2
  Row3/1 -> Mux1/3
  Mux1/1 -> Output/1
  psi/1 -> Mux/1
  Input/1 -> Mux/2

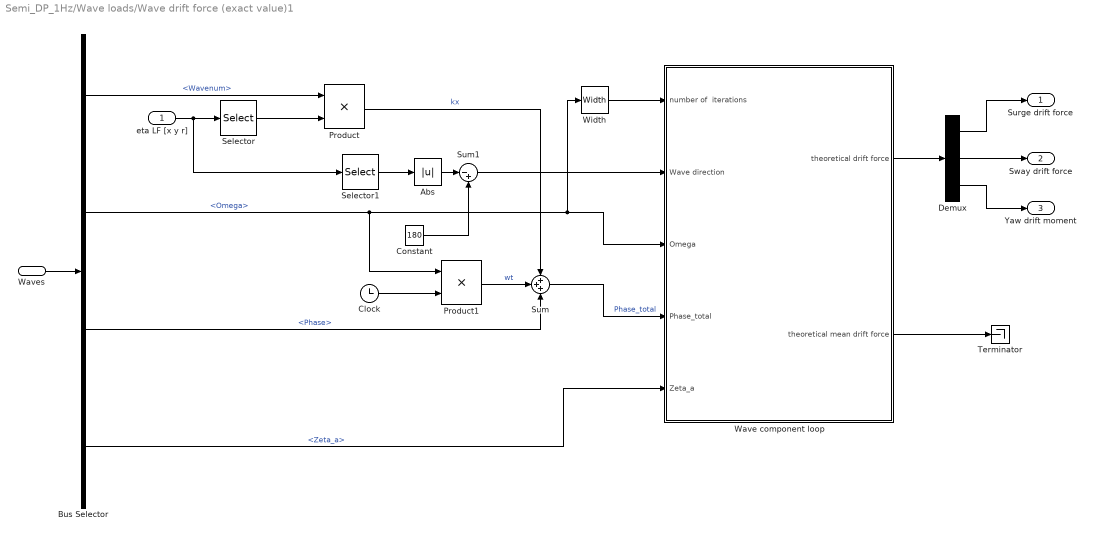
== system Semi_DP_1Hz/Wave loads/Wave drift force (exact value)1 ==
  eta LF [x y r] : Inport
  Waves : Inport  Port=2
  Abs : Abs
  Bus Selector : BusSelector  OutputSignals=Wavenum,Omega,Phase,Zeta_a
  Clock : Clock
  Constant : Constant  Value=180
  Demux : Demux  Outputs=3
  Product : Product  Inputs=**  SaturateOnIntegerOverflow=on  OutDataTypeStr=Inherit: Same as first input
  Product1 : Product  Inputs=**  SaturateOnIntegerOverflow=on  OutDataTypeStr=Inherit: Same as first input
  Selector : Selector  InputPortWidth=3  IndexOptions=Index vector (dialog)  Indices=1  OutputSizes=1
  Selector1 : Selector  InputPortWidth=3  IndexOptions=Index vector (dialog)  Indices=3  OutputSizes=1
  Sum : Sum  Inputs=+++  SaturateOnIntegerOverflow=on
  Sum1 : Sum  Inputs=|-+
  Terminator : Terminator
  Wave component loop : Subsystem  TreatAsAtomicUnit=on
  Width : Width  DataType=int32
  Surge drift force : Outport
  Sway drift force : Outport  Port=2
  Yaw drift moment : Outport  Port=3
  wires:
  Wave component loop/1(theoretical drift force) -> Demux/1
  Demux/3 -> Yaw drift moment/1
  Demux/2 -> Sway drift force/1
  Demux/1 -> Surge drift force/1
  Wave component loop/2(theoretical mean drift force) -> Terminator/1
  Sum1/1 -> Wave component loop/2(Wave direction)
  Selector1/1 -> Abs/1
  Constant/1 -> Sum1/2
  eta LF [x y r]/1 -> Selector1/1, Selector/1
  Bus Selector/1 -> Product/1  "<Wavenum>"
  Selector/1 -> Product/2
  Bus Selector/3 -> Sum/3  "<Phase>"
  Waves/1 -> Bus Selector/1
  Product1/1 -> Sum/2  "wt"
  Clock/1 -> Product1/2
  Bus Selector/2 -> Width/1, Wave component loop/3(Omega), Product1/1  "<Omega>"
  Sum/1 -> Wave component loop/4(Phase_total)  "Phase_total"
  Bus Selector/4 -> Wave component loop/5(Zeta_a)  "<Zeta_a>"
  Width/1 -> Wave component loop/1(number of  iterations)
  Product/1 -> Sum/1  "kx"
  Abs/1 -> Sum1/1

== system Semi_DP_1Hz/Wave loads/Wave elevation ==
  eta LF [x y r] : Inport
  Waves : Inport  Port=2
  Bus Selector : BusSelector  OutputSignals=Wavenum,Omega,Phase,Zeta_a
  Clock : Clock
  Product1 : Product  Inputs=**  SaturateOnIntegerOverflow=on  OutDataTypeStr=Inherit: Same as first input
  Product2 : Product  Inputs=**  SaturateOnIntegerOverflow=on  OutDataTypeStr=Inherit: Same as first input
  Selector : Selector  InputPortWidth=3  IndexOptions=Index vector (dialog)  Indices=1  OutputSizes=1
  Sum : Sum  Inputs=+++  SaturateOnIntegerOverflow=on
  Sum1 : Sum  Inputs=1  SaturateOnIntegerOverflow=on
  cos(wt+kx+phase) : Trigonometry  Operator=cos
  zeta : Product  Inputs=**  SaturateOnIntegerOverflow=on  OutDataTypeStr=Inherit: Same as first input
  Zeta(t) : Outport
  wires:
  Selector/1 -> Product2/1
  eta LF [x y r]/1 -> Selector/1
  Bus Selector/1 -> Product2/2  "<Wavenum>"
  Bus Selector/4 -> zeta/2  "<Zeta_a>"
  Bus Selector/3 -> Sum/3  "<Phase>"
  Bus Selector/2 -> Product1/1  "<Omega>"
  Waves/1 -> Bus Selector/1
  Product2/1 -> Sum/1  "kx"
  zeta/1 -> Sum1/1
  cos(wt+kx+phase)/1 -> zeta/1
  Sum/1 -> cos(wt+kx+phase)/1
  Product1/1 -> Sum/2  "wt"
  Sum1/1 -> Zeta(t)/1
  Clock/1 -> Product1/2

== system Semi_DP_1Hz/Wave loads/Wave parameters ==
  Bus Creator : BusCreator  Inputs=4
  Omega : Constant  Value=Omega
  Phase : Constant  Value=Phase
  Wavenum : Constant  Value=Wavenum
  Zeta_a : Constant  Value=Zeta_a
  Waves : Outport
  wires:
  Phase/1 -> Bus Creator/4  "Phase"
  Omega/1 -> Bus Creator/1  "Omega"
  Bus Creator/1 -> Waves/1
  Zeta_a/1 -> Bus Creator/2  "Zeta_a"
  Wavenum/1 -> Bus Creator/3  "Wavenum"

== system Semi_DP_1Hz/Wave loads/alpha-beta filter ==
  input : Inport
  Level-2 MATLAB S-Function : M-S-Function  FunctionName=msfunAB  Parameters=a,b  mask{a=a, b=b}
      mask prompts: a "alpha"; b "beta"
  output : Outport
  wires:
  input/1 -> Level-2 MATLAB S-Function/1
  Level-2 MATLAB S-Function/1 -> output/1

== system Semi_DP_1Hz/Wave loads/ideal estimation of drift force  ==
  Wave elevation : Inport
  eta LF [x y r] : Inport  Port=2
  Constant : Constant  Value=2
  Demux : Demux  Outputs=3
  Math Function : Math  Operator=pow  SaturateOnIntegerOverflow=on
  P_mean_calc : Subsystem
  Product : Product  Inputs=3  RndMeth=Zero
  surge drift force : Outport
  sway drift force : Outport  Port=2
  yaw drift moment : Outport  Port=3
  wires:
  Demux/3 -> yaw drift moment/1
  Demux/2 -> sway drift force/1
  Demux/1 -> surge drift force/1
  Product/1 -> Demux/1
  eta LF [x y r]/1 -> P_mean_calc/1(eta LF [x y r])
  Math Function/1 -> Product/2
  P_mean_calc/1(P_mean [1 2 6]) -> Product/1
  Wave elevation/1 -> Math Function/1
  Constant/1 -> Product/3, Math Function/2

== system Semi_DP_1Hz/Semi/Coriolis and centripetal forces/Subsystem ==
  v : Inport
  r : Inport  Port=2
  -a22 : Gain  Gain=-M(2,2)-Ma(2,2)  Multiplication=Matrix(K*u)  SaturateOnIntegerOverflow=on  OutDataTypeStr=Inherit: Same as input  ParamDataTypeStr=Inherit: Same as input
  -a26 : Gain  Gain=-M(2,3)-Ma(2,3)  Multiplication=Matrix(K*u)  SaturateOnIntegerOverflow=on  OutDataTypeStr=Inherit: Same as input  ParamDataTypeStr=Inherit: Same as input
  Add : Sum
  Math Function : Math  Operator=magnitude^2  SaturateOnIntegerOverflow=on
  Product : Product  RndMeth=Zero
  x direction : Outport
  wires:
  v/1 -> Product/1
  r/1 -> Product/2, Math Function/1
  Product/1 -> -a22/1
  Math Function/1 -> -a26/1
  -a22/1 -> Add/1
  -a26/1 -> Add/2
  Add/1 -> x direction/1

== system Semi_DP_1Hz/Semi/Coriolis and centripetal forces/Subsystem1 ==
  u : Inport
  r : Inport  Port=2
  Product : Product  RndMeth=Zero
  a11 : Gain  Gain=M(1,1)+Ma(1,1)  Multiplication=Matrix(K*u)  SaturateOnIntegerOverflow=on  OutDataTypeStr=Inherit: Same as input  ParamDataTypeStr=Inherit: Same as input
  y direction : Outport
  wires:
  Product/1 -> a11/1
  r/1 -> Product/2
  u/1 -> Product/1
  a11/1 -> y direction/1

== system Semi_DP_1Hz/Semi/Coriolis and centripetal forces/Subsystem2 ==
  u : Inport
  v : Inport  Port=2
  r : Inport  Port=3
  Add : Sum
  Add1 : Sum  Inputs=+-
  Product : Product  RndMeth=Zero
  Product1 : Product  RndMeth=Zero
  a11 : Gain  Gain=M(1,1)+Ma(1,1)  Multiplication=Matrix(K*u)  SaturateOnIntegerOverflow=on  OutDataTypeStr=Inherit: Same as input  ParamDataTypeStr=Inherit: Same as input
  a22 : Gain  Gain=M(2,2)+Ma(2,2)  Multiplication=Matrix(K*u)  SaturateOnIntegerOverflow=on  OutDataTypeStr=Inherit: Same as input  ParamDataTypeStr=Inherit: Same as input
  a62 : Gain  Gain=M(3,2)+Ma(3,2)  Multiplication=Matrix(K*u)  SaturateOnIntegerOverflow=on  OutDataTypeStr=Inherit: Same as input  ParamDataTypeStr=Inherit: Same as input
  yaw direction : Outport
  wires:
  u/1 -> Product/1, Product1/1
  r/1 -> Product/2
  Product/1 -> a62/1
  v/1 -> Product1/2
  Product1/1 -> a22/1, a11/1
  a22/1 -> Add1/1
  a11/1 -> Add1/2
  Add1/1 -> Add/2
  a62/1 -> Add/1
  Add/1 -> yaw direction/1

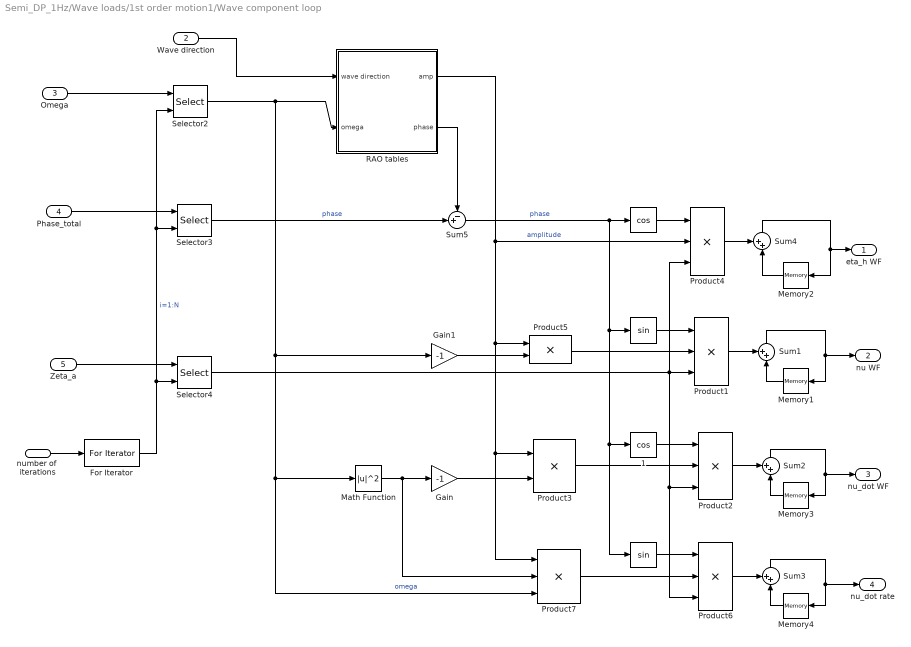
== system Semi_DP_1Hz/Wave loads/1st order motion1/Wave component loop ==
  number of  iterations : Inport
  Wave direction : Inport  Port=2
  Omega : Inport  Port=3
  Phase_total : Inport  Port=4
  Zeta_a : Inport  Port=5
  " " : Trigonometry
  "              " : Trigonometry
  "                " : Trigonometry  Operator=cos
  "                1" : Trigonometry  Operator=cos
  For Iterator : ForIterator  ResetStates=reset  IterationSource=external  IterationVariableDataType=double
  Gain : Gain  Gain=-1  SaturateOnIntegerOverflow=on  OutDataTypeStr=Inherit: Same as input  ParamDataTypeStr=Inherit: Same as input
  Gain1 : Gain  Gain=-1  SaturateOnIntegerOverflow=on  OutDataTypeStr=Inherit: Same as input  ParamDataTypeStr=Inherit: Same as input
  Math Function : Math  Operator=magnitude^2  SaturateOnIntegerOverflow=on
  Memory{1..4} (4 alike) : Memory  X0=[0 0 0 0 0 0]'  InheritSampleTime=on
  Product{1..2,4,6} (4 alike) : Product  Inputs=3  SaturateOnIntegerOverflow=on  OutDataTypeStr=Inherit: Same as first input
  Product3 : Product  Inputs=**  SaturateOnIntegerOverflow=on  OutDataTypeStr=Inherit: Same as first input
  Product5 : Product  Inputs=**  SaturateOnIntegerOverflow=on  OutDataTypeStr=Inherit: Same as first input
  Product7 : Product  Inputs=***  SaturateOnIntegerOverflow=on  OutDataTypeStr=Inherit: Same as first input
  RAO tables : Subsystem
  Selector2 : Selector  IndexOptions=Index vector (port)  Indices=[1 3]  OutputSizes=1
  Selector3 : Selector  IndexOptions=Index vector (port)  Indices=[1 3]  OutputSizes=1
  Selector4 : Selector  IndexOptions=Index vector (port)  Indices=[1 3]  OutputSizes=1
  Sum{1..4} (4 alike) : Sum  Inputs=++|  SaturateOnIntegerOverflow=on
  Sum5 : Sum  Inputs=-+|  SaturateOnIntegerOverflow=on
  eta_h WF : Outport
  nu WF : Outport  Port=2
  nu_dot WF : Outport  Port=3
  nu_dot rate : Outport  Port=4
  wires:
  RAO tables/2(phase) -> Sum5/1
  Product7/1 -> Product6/2
  " "/1 -> Product6/1
  Gain1/1 -> Product5/2
  Wave direction/1 -> RAO tables/1(wave direction)
  Memory4/1 -> Sum3/2
  Product6/1 -> Sum3/1
  Sum3/1 -> Memory4/1, nu_dot rate/1
  Selector2/1 -> Gain1/1, Product7/3, Math Function/1, RAO tables/2(omega)  "omega"
  Selector3/1 -> Sum5/2  "phase"
  Product4/1 -> Sum4/1
  Memory2/1 -> Sum4/2
  Sum4/1 -> eta_h WF/1, Memory2/1
  number of  iterations/1 -> For Iterator/1
  Omega/1 -> Selector2/1
  For Iterator/1 -> Selector2/2, Selector3/2, Selector4/2  "i=1:N"
  RAO tables/1(amp) -> Product4/2, Product7/1, Product3/1, Product5/1  "amplitude"
  Phase_total/1 -> Selector3/1
  Zeta_a/1 -> Selector4/1
  Sum5/1 -> "                "/1, " "/1, "                1"/1, "              "/1  "phase"
  "                "/1 -> Product4/1
  Selector4/1 -> Product6/3, Product2/3, Product1/3, Product4/3
  "              "/1 -> Product1/1
  Memory1/1 -> Sum1/2
  Sum1/1 -> nu WF/1, Memory1/1
  Product1/1 -> Sum1/1
  Memory3/1 -> Sum2/2
  Product2/1 -> Sum2/1
  Sum2/1 -> nu_dot WF/1, Memory3/1
  "                1"/1 -> Product2/1
  Math Function/1 -> Product7/2, Gain/1
  Gain/1 -> Product3/2
  Product3/1 -> Product2/2
  Product5/1 -> Product1/2

== system Semi_DP_1Hz/Wave loads/Wave drift force (exact value)1/Wave component loop ==
  number of  iterations : Inport
  Wave direction : Inport  Port=2
  Omega : Inport  Port=3
  Phase_total : Inport  Port=4
  Zeta_a : Inport  Port=5
  Add : Sum
  calculation of theoredtical mean drift force : Subsystem
  calculation of theoretical slowly varying drift force : Subsystem  TreatAsAtomicUnit=on
  theoretical drift force : Outport
  theoretical mean drift force : Outport  Port=2
  wires:
  Add/1 -> theoretical drift force/1
  calculation of theoretical slowly varying drift force/1(theoretical S_V drift force) -> Add/2
  Phase_total/1 -> calculation of theoretical slowly varying drift force/5(Phase_total)
  calculation of theoredtical mean drift force/1(theoretical mean drift force) -> theoretical mean drift force/1, Add/1
  Zeta_a/1 -> calculation of theoretical slowly varying drift force/4(Zeta_a), calculation of theoredtical mean drift force/3(Zeta_a)
  Omega/1 -> calculation of theoretical slowly varying drift force/3(Omega), calculation of theoredtical mean drift force/2(Omega)
  Wave direction/1 -> calculation of theoretical slowly varying drift force/2(Wave direction), calculation of theoredtical mean drift force/1(Wave direction)
  number of  iterations/1 -> calculation of theoretical slowly varying drift force/1(number of  iterations), calculation of theoredtical mean drift force/4(number of  iterations)

== system Semi_DP_1Hz/Wave loads/ideal estimation of drift force /P_mean_calc ==
  eta LF [x y r] : Inport
  Abs : Abs
  Constant : Constant  Value=180
  Lookup Table (n-D) : Lookup_n-D  NumberOfTableDimensions=1  BreakpointsForDimension1=QTF_Dir  Table=P_mean(:,1)  DiagnosticForOutOfRangeInput=Warning  InputSameDT=on
  Lookup Table (n-D)1 : Lookup_n-D  NumberOfTableDimensions=1  BreakpointsForDimension1=QTF_Dir  Table=P_mean(:,2)  DiagnosticForOutOfRangeInput=Warning  InputSameDT=on
  Lookup Table (n-D)2 : Lookup_n-D  NumberOfTableDimensions=1  BreakpointsForDimension1=QTF_Dir  Table=P_mean(:,3)  DiagnosticForOutOfRangeInput=Warning  InputSameDT=on
  Lookup Table (n-D)3 : Lookup_n-D  NumberOfTableDimensions=1  BreakpointsForDimension1=QTF_Dir  Table=P_mean(:,4)  DiagnosticForOutOfRangeInput=Warning  InputSameDT=on
  Lookup Table (n-D)4 : Lookup_n-D  NumberOfTableDimensions=1  BreakpointsForDimension1=QTF_Dir  Table=P_mean(:,5)  DiagnosticForOutOfRangeInput=Warning  InputSameDT=on
  Lookup Table (n-D)5 : Lookup_n-D  NumberOfTableDimensions=1  BreakpointsForDimension1=QTF_Dir  Table=P_mean(:,6)  DiagnosticForOutOfRangeInput=Warning  InputSameDT=on
  Mux : Mux  Inputs=3
  Mux1 : Mux  Inputs=3
  Selector1 : Selector  InputPortWidth=3  IndexOptions=Index vector (dialog)  Indices=3  OutputSizes=1
  Sum1 : Sum  Inputs=|-+
  Terminator : Terminator
  P_mean [1 2 6] : Outport
  wires:
  Mux/1 -> P_mean [1 2 6]/1
  Mux1/1 -> Terminator/1
  Lookup Table (n-D)4/1 -> Mux1/3
  Lookup Table (n-D)3/1 -> Mux1/2
  Lookup Table (n-D)2/1 -> Mux1/1
  Lookup Table (n-D)5/1 -> Mux/3
  Lookup Table (n-D)1/1 -> Mux/2
  Lookup Table (n-D)/1 -> Mux/1
  Sum1/1 -> Lookup Table (n-D)5/1, Lookup Table (n-D)4/1, Lookup Table (n-D)3/1, Lookup Table (n-D)2/1, Lookup Table (n-D)1/1, Lookup Table (n-D)/1
  eta LF [x y r]/1 -> Selector1/1
  Constant/1 -> Sum1/2
  Abs/1 -> Sum1/1
  Selector1/1 -> Abs/1
